simulink model "BLE_angle_control_R2024b"  (R2024b)
settings: Solver=FixedStepDiscrete  StartTime=0.0  StopTime=inf  FixedStep=0.005  RelTol=1e-3  EnableMultiTasking=on
undefined symbols (not defined in the file or in its folder): angle_control2, b570118e, BLE_Receive, c544, df2f, eff837991f54, fce70352
libraries: roller485lib x3, arduinolib x1
settings Model: ExtModeTrigDuration=2  Creator=kawata  LastModifiedBy=kawata
settings SolverCC: AutoInsertRateTranBlk=on
settings DataIOCC: ReturnWorkspaceOutputs=off
settings OptimizationCC: EnhancedBackFolding=on  PassReuseOutputArgsThreshold=0  MaxStackSize=64  OptimizeBlockOrder=speed  DifferentSizesBufferReuse=on  OptimizationCustomize=off
settings DebuggingCC: ParameterTunabilityLossMsg=error
settings HardwareCC: ProdBitPerPointer=32  ProdBitPerSizeT=32  ProdBitPerPtrDiffT=32  ProdLargestAtomicInteger=Long  ProdLargestAtomicFloat=Double  ProdWordSize=32  ProdHWDeviceType=ARM Compatible->ARM Cortex
settings SFSimCC: MATLABDynamicMemAlloc=off
settings RTWCC: Description=Embedded Coder  SystemTargetFile=ert.tlc  HardwareBoard=ESP32-WROOM(Arduino Compatible)  TLCOptions="-aInlineSetEventsForThisBaseRateFcn=TLC_FALSE -aSuppressMultiTaskScheduler=TLC_FALSE  -aRateBasedStepFcn=0"  TemplateMakefile=ert_default_tmf  Toolchain=ESP32  BuildConfiguration=Faster Runs
settings CodeAppCC: ForceParamTrailComments=on  OperatorAnnotations=on
settings ERTTargetCC: ERTCustomFileBanners=off  SupportContinuousTime=on  SupportNonInlinedSFcns=on  RemoveResetFunc=off  SupportVariableSizeSignals=on  ModelStepFunctionPrototypeControlCompliant=off  ExtModeTransport=3  ExtModeStaticAlloc=on  ExtModeAutomaticAllocSize=off  ExtModeStaticAllocSize=65536  ExtModeMexFile=ext_xcp  ExtModeIntrfLevel=Level2 - Open  InlinedParameterPlacement=Hierarchical  DynamicArrayContainerType=coder::array

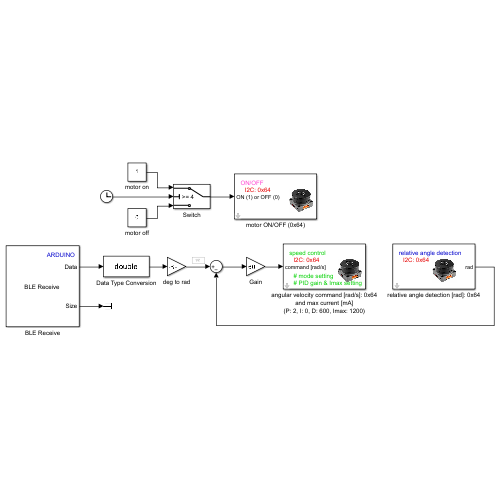
[thumbnail: Simulink's stored preview of the top-level diagram]
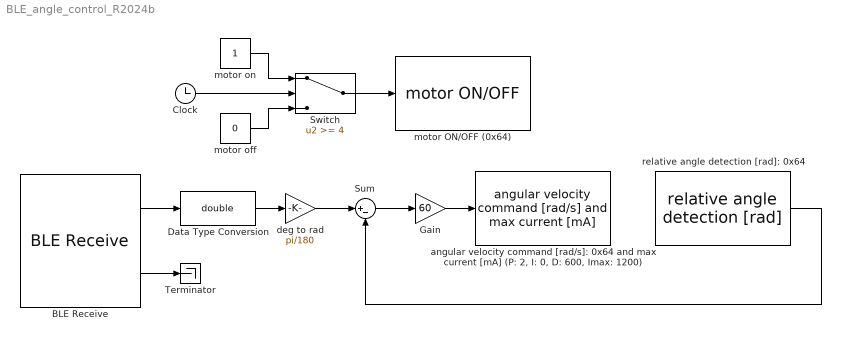
== system BLE_angle_control_R2024b ==
  BLE Receive : arduinolib/BLE Receive  DeviceMode=Peripheral (Server)  BluetoothAddress=""  CharUUID=""  ServiceUUID=""  device=No Devices  character=No Characteristics  CustomService=on  ServiceName=Generic Access  CharacteristicName=Device Name  CustomServiceUUID=fce70352-c544-48f4-9760-7568263b7922  CustomCharUUID=b570118e-df2f-4545-9cf9-eff837991f54  DataSize=1  SampleTime=0.1  charseruuid=<empty>  seruuid=00001810-0000-1000-8000-00805f9b34fb  PeripheralService=00001800-0000-1000-8000-00805f9b34fb  PeripheralCharacteristic=00002a00-0000-1000-8000-00805f9b34fb  chruuid=00002a00-0000-1000-8000-00805f9b34fb  BLEId=angle_control2/BLE_Receive  Devicename=""  IsCustomService=0
      settings: SourceProductName=Common
  Clock : Clock
  Data Type Conversion : DataTypeConversion  OutDataTypeStr=double  SaturateOnIntegerOverflow=off  RndMeth=Floor
  Gain : Gain  Gain=60
  Sum : Sum  Inputs=|+-
  Switch : Switch  Threshold=4  SaturateOnIntegerOverflow=off  InputSameDT=off
  Terminator : Terminator
  "angular velocity command [rad/s]: 0x64 and max current [mA] (P: 2, I: 0, D: 600, Imax: 1200)" : roller485lib/I2C Write/angular velocity command [rad//s] and max current [mA]  I2CAddress=0x64  set_time=3  speed_P=2  speed_I=0  speed_D=600  max_current=1200
      settings: SourceProductName=Roller485 Library
  deg to rad : Gain  Gain=pi/180
  motor ON/OFF (0x64) : roller485lib/motor ON//OFF  I2CAddress=0x64
      settings: SourceProductName=Roller485 Library
  motor off : Constant  Value=0
  motor on : Constant
  relative angle detection [rad]: 0x64 : roller485lib/I2C Read/relative angle detection [rad]  I2CAddress=0x64  sample_time=0.005
      settings: SourceProductName=Roller485 Library
  wires:
  motor on/1 -> Switch/1
  Clock/1 -> Switch/2
  motor off/1 -> Switch/3
  Switch/1 -> motor ON/OFF (0x64)/1
  Gain/1 -> "angular velocity command [rad/s]: 0x64 and max current [mA] (P: 2, I: 0, D: 600, Imax: 1200)"/1
  Sum/1 -> Gain/1
  relative angle detection [rad]: 0x64/1 -> Sum/2
  deg to rad/1 -> Sum/1
  BLE Receive/2 -> Terminator/1
  Data Type Conversion/1 -> deg to rad/1
  BLE Receive/1 -> Data Type Conversion/1
